simulink model "heli_q81"  (R2015b)
settings: Solver=ode1  StartTime=0.0  StopTime=inf  FixedStep=0.002  RelTol=1e-3
PostLoadFcn:
  | qc_set_target_type(getConfigSet(bdroot, 'QUARC Default Target Configuration'));
values from neighbouring files (symbols this model uses):
  F = inv(C*inv(B*K-A)*B)    [init_heli.m]
  F_aug = inv(C*inv(B*K_aug_K1-A)*B)    [init_heli.m]
  Joystick_gain_x = 1    [init_heli.m]
  Joystick_gain_y = 1    [init_heli.m]
  K = lqr(A,B,Q,R)    [init_heli.m]
  K_aug = lqr(A_aug,B_aug,Q_aug,R_aug)    [init_heli.m]
  v_s0 = 7.7    [init_heli.m]
undefined symbols (not defined in the file or in its folder): HIL, qc_get_step_size
libraries: quarc_library x4
settings Model: SimulationMode=external  ExtModeTrigDuration=5000  Creator=Rchan  LastModifiedBy=sanderfu
settings SolverCC: PositivePriorityOrder=on
settings DataIOCC: SaveFormat=Array  SignalLoggingSaveFormat=ModelDataLogs
settings OptimizationCC: ExpressionDepthLimit=2147483647  InitFltsAndDblsToZero=on
settings DebuggingCC: SaveWithParameterizedLinksMsg=none  UnderspecifiedInitializationDetection=Classic  MergeDetectMultiDrivingBlocksExec=none  SolverPrmCheckMsg=warning  MultiTaskDSMMsg=warning  MultiTaskCondExecSysMsg=none  FcnCallInpInsideContextMsg=UseLocalSettings  StateNameClashWarn=warning
settings HardwareCC: ProdBitPerPointer=32  ProdLargestAtomicFloat=None  ProdIntDivRoundTo=Undefined  ProdEndianess=Unspecified  ProdWordSize=32  ProdHWDeviceType=32-bit Generic
settings RTWCC: SystemTargetFile=quarc_win64.tlc  TemplateMakefile=quarc_default_tmf  Description=QUARC Win64 Target
settings GRTTargetCC: ParMdlRefBuildCompliant=off  CompOptLevelCompliant=off  GeneratePreprocessorConditionals=Disable all  CombineOutputUpdateFcns=off  MatFileLogging=off  GRTInterface=on  UseToolchainInfoCompliant=off  ExtMode=on  ExtModeMexFile=quarc_comm
settings ConfigComp: CovModelRefEnable=Off  CovSFcnEnable=off

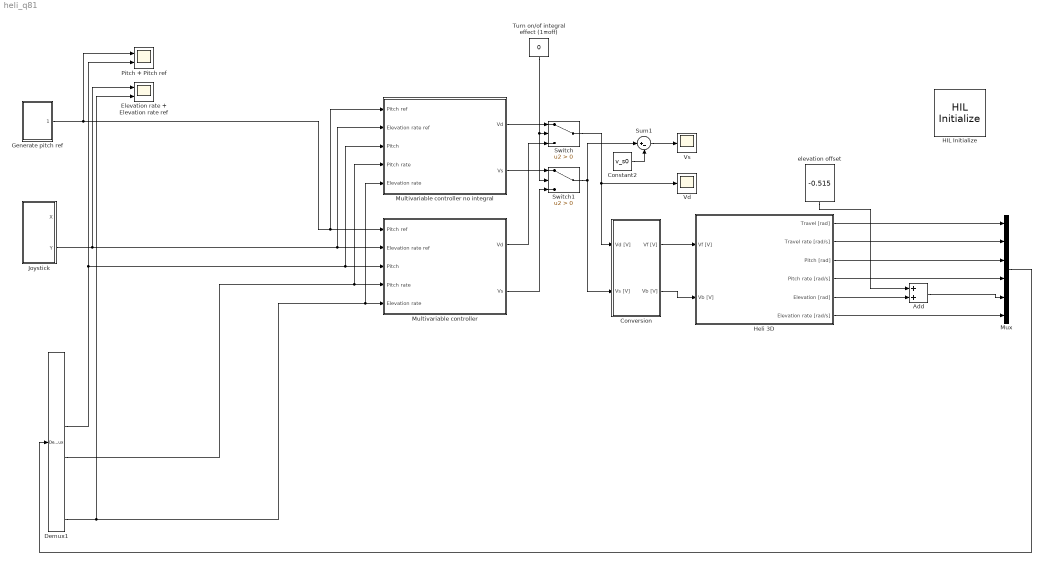
== system heli_q81 ==
  Add : Sum
  Constant2 : Constant  Value=v_s0
  Conversion : Subsystem
  Demux1 : Demux  Outputs=6
  Elevation rate + Elevation rate ref : Scope  NumInputPorts=2
  Generate pitch ref : Subsystem
  HIL Initialize : quarc_library/Data Acquisition/Generic/Configuration/HIL Initialize  Priority=-99  object_name=HIL-1  board_type=q8_usb  board_number=0  board_options=update_rate=normal;decimation=1  exclusive=off  active=off  hardware_clocks=[0:2]  clock_modes=[]  initial_clock_frequencies=[]  set_clock_params_at_start=off  set_clock_params_at_switch_in=off  set_clock_frequencies_at_start=off  set_clock_frequencies_at_switch_in=off  analog_input_channels=[0:7]  analog_input_maximums=10  analog_input_minimums=-10  set_analog_input_params_at_start=on  set_analog_input_params_at_switch_in=off  analog_output_channels=[0:7]  analog_output_maximums=10  analog_output_minimums=-10  initial_analog_outputs=[0]  final_analog_outputs=[0]  watchdog_analog_outputs=0  set_analog_output_params_at_start=on  set_analog_output_params_at_switch_in=off  set_analog_outputs_at_start=on  set_analog_outputs_at_switch_in=off  set_analog_outputs_at_terminate=on  set_analog_outputs_at_switch_out=off  set_analog_outputs_on_watchdog=off  digital_input_channels=[]  digital_output_channels=[]  digital_output_configuration=[]  initial_digital_outputs=[1]  final_digital_outputs=[1]  watchdog_digital_outputs=[1]  set_digital_output_params_at_start=off  set_digital_output_params_at_switch_in=off  set_digital_outputs_at_start=on  set_digital_outputs_at_switch_in=off  set_digital_outputs_at_terminate=on  set_digital_outputs_at_switch_out=off  set_digital_outputs_on_watchdog=off  encoder_channels=[0:7]  quadrature=[4]  encoder_filter_frequency=[]  initial_encoder_counts=[0]  set_encoder_params_at_start=on  set_encoder_params_at_switch_in=off  set_encoder_counts_at_start=on  set_encoder_counts_at_switch_in=off  pwm_channels=[0:7]  pwm_modes=0  pwm_frequency=99.532799999999995e6/4095  pwm_configuration=[0]  pwm_alignment=[0]  pwm_polarity=[1]  pwm_leading_deadband=[0]  pwm_trailing_deadband=[0]  initial_pwm_outputs=[0]  final_pwm_outputs=[0]  watchdog_pwm_outputs=[0]  set_pwm_params_at_start=on  set_pwm_params_at_switch_in=off  set_pwm_outputs_at_start=on  set_pwm_outputs_at_switch_in=off  set_pwm_outputs_at_terminate=on  set_pwm_outputs_at_switch_out=off  set_pwm_outputs_on_watchdog=off  other_output_channels=[]  initial_other_outputs=[]  final_other_outputs=[]  watchdog_other_outputs=[]  set_other_outputs_at_start=off  set_other_outputs_at_switch_in=off  set_other_outputs_at_terminate=off  set_other_outputs_at_switch_out=off  set_other_outputs_on_watchdog=off
  Heli 3D : Subsystem
  Joystick : Subsystem
  Multivariable controller : Subsystem
  Multivariable controller no integral : Subsystem
  Mux : Mux  Inputs=6
  Pitch + Pitch ref : Scope  NumInputPorts=2
  Sum1 : Sum  Inputs=|+-
  Switch : Switch  Criteria=u2 > Threshold
  Switch1 : Switch  Criteria=u2 > Threshold
  Turn on/of integral effect (1=off) : Constant  Value=0
  Vd : Scope
  Vs : Scope
  elevation offset : Constant  Value=-0.515
  wires:
  Heli 3D/1(Travel [rad]) -> Mux/1
  Heli 3D/2(Travel rate [rad/s]) -> Mux/2
  Heli 3D/3(Pitch [rad]) -> Mux/3
  Heli 3D/4(Pitch rate [rad/s]) -> Mux/4
  Heli 3D/5(Elevation [rad]) -> Add/2
  Heli 3D/6(Elevation rate [rad/s]) -> Mux/6
  Add/1 -> Mux/5
  elevation offset/1 -> Add/1
  Joystick/2(Y) -> Multivariable controller no integral/2(Elevation rate ref), Multivariable controller/2(Elevation rate ref), Elevation rate + Elevation rate ref/1
  Mux/1 -> Demux1/1
  Demux1/3 -> Multivariable controller no integral/3(Pitch), Multivariable controller/3(Pitch), Pitch + Pitch ref/2
  Multivariable controller/1(Vd) -> Switch/3
  Multivariable controller/2(Vs) -> Switch1/3
  Generate pitch ref/1(Pitch ref) -> Multivariable controller no integral/1("Pitch ref "), Multivariable controller/1("Pitch ref "), Pitch + Pitch ref/1
  Demux1/4 -> Multivariable controller no integral/4(Pitch rate), Multivariable controller/4(Pitch rate)
  Demux1/6 -> Multivariable controller no integral/5(Elevation rate), Multivariable controller/5(Elevation rate), Elevation rate + Elevation rate ref/2
  Multivariable controller no integral/1(Vd) -> Switch/1
  Multivariable controller no integral/2(Vs) -> Switch1/1
  Turn on/of integral effect (1=off)/1 -> Switch1/2, Switch/2
  Switch1/1 -> Sum1/1, Conversion/2(Vs [V])
  Switch/1 -> Vd/1, Conversion/1(Vd [V])
  Sum1/1 -> Vs/1
  Constant2/1 -> Sum1/2
  Conversion/1(Vf [V]) -> Heli 3D/1(Vf [V])
  Conversion/2(Vb [V]) -> Heli 3D/2(Vb [V])

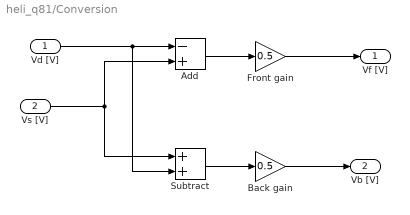
== system heli_q81/Conversion ==
  Vd [V] : Inport
  Vs [V] : Inport  Port=2
  Add : Sum  Inputs=-+
  Back gain : Gain  Gain=0.5
  Front gain : Gain  Gain=0.5
  Subtract : Sum
  Vf [V] : Outport
  Vb [V] : Outport  Port=2
  wires:
  Vd [V]/1 -> Subtract/2, Add/1
  Vs [V]/1 -> Subtract/1, Add/2
  Subtract/1 -> Back gain/1
  Back gain/1 -> Vb [V]/1
  Add/1 -> Front gain/1
  Front gain/1 -> Vf [V]/1

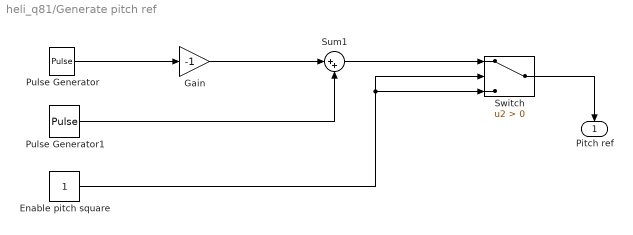
== system heli_q81/Generate pitch ref ==
  Enable pitch square : Constant
  Gain : Gain  Gain=-1
  Pulse Generator : DiscretePulseGenerator  PulseType=Time based  Amplitude=0.5  Period=20  PulseWidth=25  PhaseDelay=10
  Pulse Generator1 : DiscretePulseGenerator  PulseType=Time based  Amplitude=0.5  Period=20  PulseWidth=25  PhaseDelay=25
  Sum1 : Sum  Inputs=|++
  Switch : Switch  Criteria=u2 > Threshold
  Pitch ref : Outport
  wires:
  Enable pitch square/1 -> Switch/3, Switch/2
  Sum1/1 -> Switch/1
  Pulse Generator/1 -> Gain/1
  Gain/1 -> Sum1/1
  Pulse Generator1/1 -> Sum1/2
  Switch/1 -> Pitch ref/1

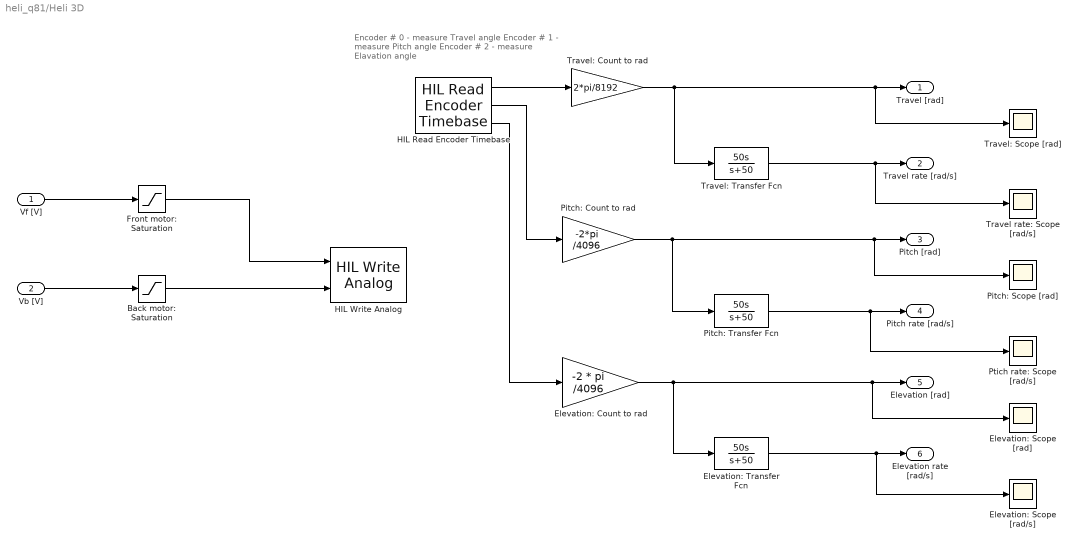
== system heli_q81/Heli 3D ==
  note: Encoder # 0 - measure Travel angle
      | Encoder # 1 - measure Pitch angle
      | Encoder # 2 - measure Elavation angle
  Vf [V] : Inport
  Vb [V] : Inport  Port=2
  Back motor: Saturation : Saturate  UpperLimit=5  LowerLimit=-5
  Elevation: Count to rad : Gain  Gain=-2 * pi /4096
  Elevation: Scope [rad/s] : Scope
  Elevation: Scope [rad] : Scope
  Elevation: Transfer Fcn : TransferFcn  Numerator=[50 0]  Denominator=[1 50]
  Front motor: Saturation : Saturate  UpperLimit=5  LowerLimit=-5
  HIL Read Encoder Timebase : quarc_library/Data Acquisition/Generic/Timebases/HIL Read Encoder Timebase  object_name=HIL-1  clock=0  channels=[0:2]  samples_in_buffer=max(ceil(1/qc_get_step_size), 1)  active=on  vector_output=off  data_type_mode=Inherit via back propagation  data_type=double
  HIL Write Analog : quarc_library/Data Acquisition/Generic/Immediate I//O/HIL Write Analog  object_name=HIL-1  channels=[0:1]  sample_time=-1  active=off  vector_input=off
  Pitch: Count to rad : Gain  Gain=-2*pi /4096
  Pitch: Scope [rad] : Scope
  Pitch: Transfer Fcn : TransferFcn  Numerator=[50 0]  Denominator=[1 50]
  Ptich rate: Scope [rad/s] : Scope
  Travel rate: Scope [rad/s] : Scope
  Travel: Count to rad : Gain  Gain=2*pi/8192
  Travel: Scope [rad] : Scope
  Travel: Transfer Fcn : TransferFcn  Numerator=[50 0]  Denominator=[1 50]
  Travel [rad] : Outport
  Travel rate [rad/s] : Outport  Port=2
  Pitch [rad] : Outport  Port=3
  Pitch rate [rad/s] : Outport  Port=4
  Elevation [rad] : Outport  Port=5
  Elevation rate [rad/s] : Outport  Port=6
  wires:
  HIL Read Encoder Timebase/1 -> Travel: Count to rad/1
  HIL Read Encoder Timebase/2 -> Pitch: Count to rad/1
  HIL Read Encoder Timebase/3 -> Elevation: Count to rad/1
  Travel: Count to rad/1 -> Travel: Scope [rad]/1, Travel [rad]/1, Travel: Transfer Fcn/1
  Travel: Transfer Fcn/1 -> Travel rate: Scope [rad/s]/1, Travel rate [rad/s]/1
  Pitch: Count to rad/1 -> Pitch: Transfer Fcn/1, Pitch: Scope [rad]/1, Pitch [rad]/1
  Pitch: Transfer Fcn/1 -> Ptich rate: Scope [rad/s]/1, Pitch rate [rad/s]/1
  Elevation: Count to rad/1 -> Elevation: Transfer Fcn/1, Elevation: Scope [rad]/1, Elevation [rad]/1
  Elevation: Transfer Fcn/1 -> Elevation: Scope [rad/s]/1, Elevation rate [rad/s]/1
  Vf [V]/1 -> Front motor: Saturation/1
  Vb [V]/1 -> Back motor: Saturation/1
  Front motor: Saturation/1 -> HIL Write Analog/1
  Back motor: Saturation/1 -> HIL Write Analog/2

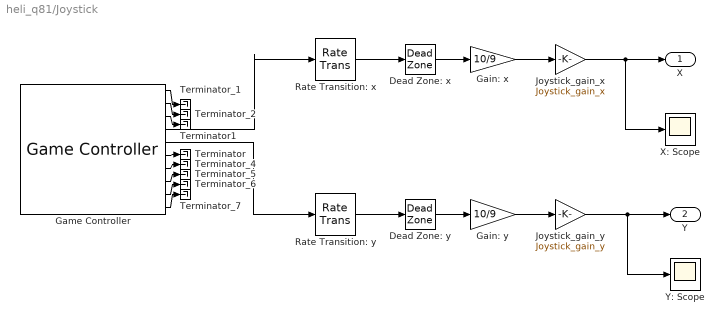
== system heli_q81/Joystick ==
  Dead Zone: x : DeadZone  LowerValue=-0.1  UpperValue=0.1  SaturateOnIntegerOverflow=on
  Dead Zone: y : DeadZone  LowerValue=-0.1  UpperValue=0.1  SaturateOnIntegerOverflow=on
  Gain: x : Gain  Gain=10/9
  Gain: y : Gain  Gain=10/9
  Game Controller : quarc_library/Devices/Peripherals/Target/Game Controller  controller=1  buffer_size=12  deadzone=[]  saturation=[]  sample_time=max(qc_get_step_size, 0.01)  auto_center=off  enabled=on
  Joystick_gain_x : Gain  Gain=Joystick_gain_x
  Joystick_gain_y : Gain  Gain=Joystick_gain_y
  Rate Transition: x : RateTransition
  Rate Transition: y : RateTransition
  Terminator : Terminator
  Terminator1 : Terminator
  Terminator_{1..2,4..7} (6 alike) : Terminator
  X: Scope : Scope
  Y: Scope : Scope
  X : Outport
  Y : Outport  Port=2
  wires:
  Rate Transition: y/1 -> Dead Zone: y/1
  Rate Transition: x/1 -> Dead Zone: x/1
  Game Controller/5 -> Rate Transition: y/1
  Game Controller/4 -> Rate Transition: x/1
  Game Controller/1 -> Terminator_1/1
  Game Controller/2 -> Terminator_2/1
  Game Controller/7 -> Terminator_4/1
  Game Controller/8 -> Terminator_5/1
  Game Controller/9 -> Terminator_6/1
  Game Controller/10 -> Terminator_7/1
  Game Controller/3 -> Terminator1/1
  Game Controller/6 -> Terminator/1
  Dead Zone: x/1 -> Gain: x/1
  Dead Zone: y/1 -> Gain: y/1
  Gain: x/1 -> Joystick_gain_x/1
  Gain: y/1 -> Joystick_gain_y/1
  Joystick_gain_x/1 -> X/1, X: Scope/1
  Joystick_gain_y/1 -> Y: Scope/1, Y/1

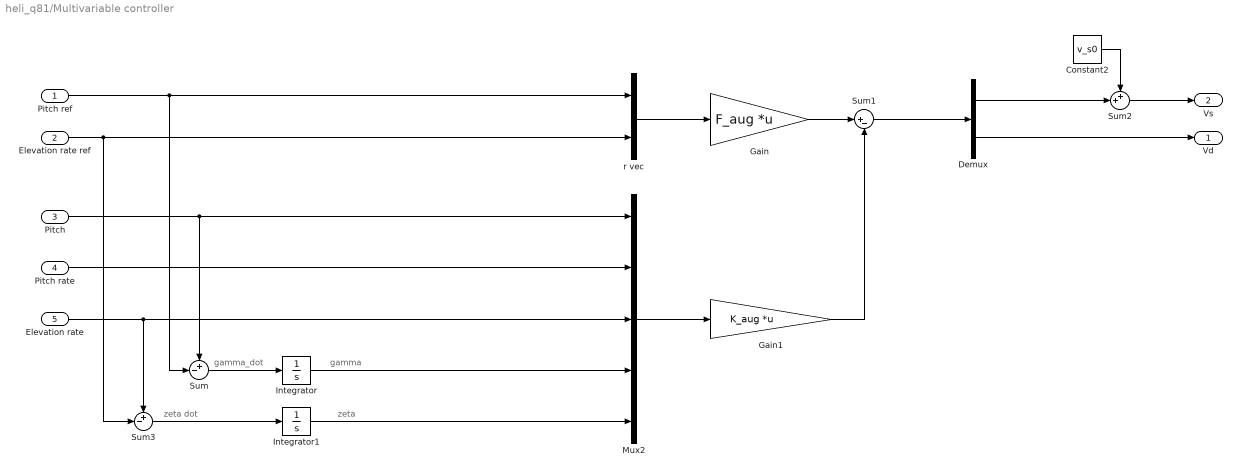
== system heli_q81/Multivariable controller ==
  note: zeta
  note: zeta dot
  note: gamma
  note: gamma_dot
  "Pitch ref " : Inport
  Elevation rate ref : Inport  Port=2
  Pitch : Inport  Port=3
  Pitch rate : Inport  Port=4
  Elevation rate : Inport  Port=5
  Constant2 : Constant  Value=v_s0
  Demux : Demux  Outputs=2
  Gain : Gain  Gain=F_aug  Multiplication=Matrix(K*u) (u vector)
  Gain1 : Gain  Gain=K_aug  Multiplication=Matrix(K*u) (u vector)
  Integrator : Integrator
  Integrator1 : Integrator
  Mux2 : Mux  Inputs=5
  Sum : Sum  Inputs=+-|
  Sum1 : Sum  Inputs=|+-
  Sum2 : Sum  Inputs=++|
  Sum3 : Sum  Inputs=+-|
  r vec : Mux  Inputs=2
  Vd : Outport
  Vs : Outport  Port=2
  wires:
  r vec/1 -> Gain/1
  Elevation rate ref/1 -> Sum3/2, r vec/2
  Gain/1 -> Sum1/1
  Mux2/1 -> Gain1/1
  Gain1/1 -> Sum1/2
  Elevation rate/1 -> Mux2/3, Sum3/1
  Pitch/1 -> Sum/1, Mux2/1
  Pitch rate/1 -> Mux2/2
  Constant2/1 -> Sum2/1
  Demux/2 -> Vd/1
  Sum2/1 -> Vs/1
  Sum1/1 -> Demux/1
  Demux/1 -> Sum2/2
  "Pitch ref "/1 -> Sum/2, r vec/1
  Sum/1 -> Integrator/1
  Sum3/1 -> Integrator1/1
  Integrator/1 -> Mux2/4
  Integrator1/1 -> Mux2/5

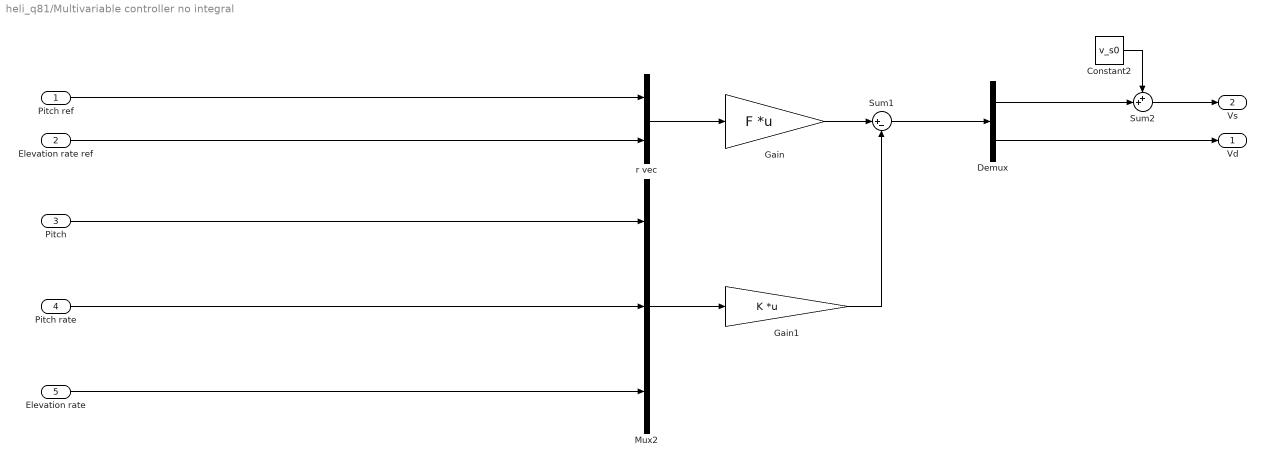
== system heli_q81/Multivariable controller no integral ==
  "Pitch ref " : Inport
  Elevation rate ref : Inport  Port=2
  Pitch : Inport  Port=3
  Pitch rate : Inport  Port=4
  Elevation rate : Inport  Port=5
  Constant2 : Constant  Value=v_s0
  Demux : Demux  Outputs=2
  Gain : Gain  Gain=F  Multiplication=Matrix(K*u) (u vector)
  Gain1 : Gain  Gain=K  Multiplication=Matrix(K*u) (u vector)
  Mux2 : Mux  Inputs=3
  Sum1 : Sum  Inputs=|+-
  Sum2 : Sum  Inputs=++|
  r vec : Mux  Inputs=2
  Vd : Outport
  Vs : Outport  Port=2
  wires:
  r vec/1 -> Gain/1
  Elevation rate ref/1 -> r vec/2
  Gain/1 -> Sum1/1
  Mux2/1 -> Gain1/1
  Gain1/1 -> Sum1/2
  Elevation rate/1 -> Mux2/3
  Pitch/1 -> Mux2/1
  Pitch rate/1 -> Mux2/2
  Constant2/1 -> Sum2/1
  Demux/2 -> Vd/1
  Sum2/1 -> Vs/1
  Sum1/1 -> Demux/1
  Demux/1 -> Sum2/2
  "Pitch ref "/1 -> r vec/1
